simulink library "MAPH"  (R2016a)
settings: Solver=ode45  StartTime=0.0  StopTime=10.0  RelTol=1e-3
undefined symbols (not defined in the file): BUSY, CLEANED, EMPTY, FORWARD, ROB_EAST, ROB_NORTH, ROB_SOUTH, ROB_WEST, ROOM_SIDE_SIZE, UNCOVERED
settings Model: Creator=oelkawok  LastModifiedBy=omaro
settings DataIOCC: LimitDataPoints=on
settings DebuggingCC: AllowSymbolicDim=off

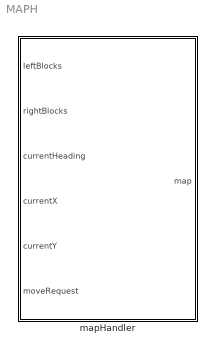
== system MAPH ==
  mapHandler : Subsystem

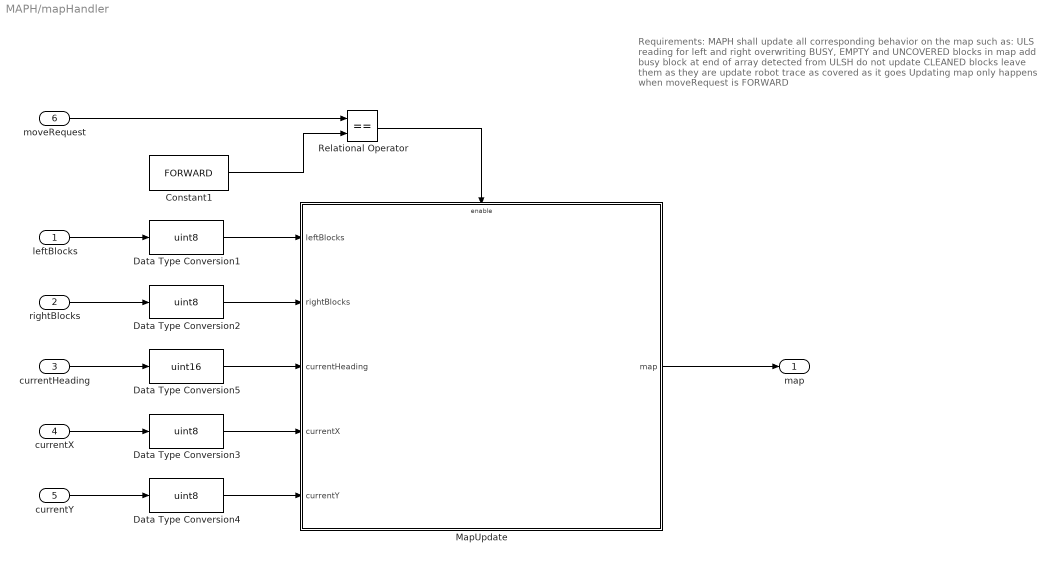
== system MAPH/mapHandler ==
  note: Requirements:
      | MAPH shall update all corresponding behavior on the map such as:
      | ULS reading for left and right
      | overwriting BUSY, EMPTY and UNCOVERED blocks in map
      | add busy block at end of array detected from ULSH
      | do not update CLEANED blocks leave them as they are
      | update robot trace as covered as it goes
      | Updating map only happens when moveRequest is FORWARD
  leftBlocks : Inport
  rightBlocks : Inport  Port=2
  currentHeading : Inport  Port=3
  currentX : Inport  Port=4
  currentY : Inport  Port=5
  moveRequest : Inport  Port=6
  Constant1 : Constant  Value=FORWARD
  Data Type Conversion{1..4} (4 alike) : DataTypeConversion  OutDataTypeStr=uint8
  Data Type Conversion5 : DataTypeConversion  OutDataTypeStr=uint16
  MapUpdate : Subsystem
  Relational Operator : RelationalOperator  Operator===  OutDataTypeStr=boolean
  map : Outport
  wires:
  Data Type Conversion1/1 -> MapUpdate/1(leftBlocks)
  Data Type Conversion2/1 -> MapUpdate/2(rightBlocks)
  Data Type Conversion3/1 -> MapUpdate/4(currentX)
  Data Type Conversion4/1 -> MapUpdate/5(currentY)
  Data Type Conversion5/1 -> MapUpdate/3(currentHeading)
  Relational Operator/1 -> MapUpdate/Enable
  moveRequest/1 -> Relational Operator/1
  Constant1/1 -> Relational Operator/2
  MapUpdate/1(map) -> map/1
  currentY/1 -> Data Type Conversion4/1
  currentX/1 -> Data Type Conversion3/1
  currentHeading/1 -> Data Type Conversion5/1
  rightBlocks/1 -> Data Type Conversion2/1
  leftBlocks/1 -> Data Type Conversion1/1

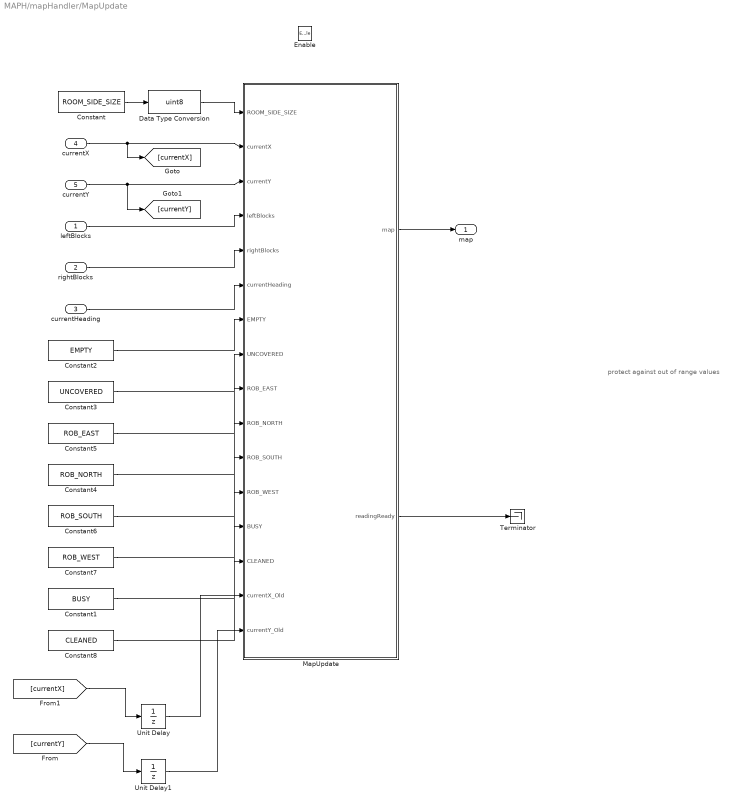
== system MAPH/mapHandler/MapUpdate ==
  note: protect against out of range values
  leftBlocks : Inport
  rightBlocks : Inport  Port=2
  currentHeading : Inport  Port=3
  currentX : Inport  Port=4
  currentY : Inport  Port=5
  Enable : EnablePort
  Constant : Constant  Value=ROOM_SIDE_SIZE
  Constant1 : Constant  Value=BUSY
  Constant2 : Constant  Value=EMPTY
  Constant3 : Constant  Value=UNCOVERED
  Constant4 : Constant  Value=ROB_NORTH
  Constant5 : Constant  Value=ROB_EAST
  Constant6 : Constant  Value=ROB_SOUTH
  Constant7 : Constant  Value=ROB_WEST
  Constant8 : Constant  Value=CLEANED
  Data Type Conversion : DataTypeConversion  OutDataTypeStr=uint8
  MapUpdate : Stateflow chart  TreatAsAtomicUnit=on
  Terminator : Terminator
  Unit Delay : UnitDelay  InitialCondition=10  SampleTime=-1
  Unit Delay1 : UnitDelay  InitialCondition=12  SampleTime=-1
  map : Outport
  wires:
  MapUpdate/1(map) -> map/1
  Unit Delay1/1 -> MapUpdate/16(currentY_Old)
  Unit Delay/1 -> MapUpdate/15(currentX_Old)
  [currentY] -> Unit Delay1/1
  [currentX] -> Unit Delay/1
  MapUpdate/2(readingReady) -> Terminator/1
  Constant2/1 -> MapUpdate/7(EMPTY)
  Constant8/1 -> MapUpdate/14(CLEANED)
  Constant3/1 -> MapUpdate/8(UNCOVERED)
  currentX/1 -> MapUpdate/2(currentX), [currentX]
  currentY/1 -> MapUpdate/3(currentY), [currentY]
  leftBlocks/1 -> MapUpdate/4(leftBlocks)
  rightBlocks/1 -> MapUpdate/5(rightBlocks)
  currentHeading/1 -> MapUpdate/6(currentHeading)
  Constant/1 -> Data Type Conversion/1
  Constant1/1 -> MapUpdate/13(BUSY)
  Data Type Conversion/1 -> MapUpdate/1(ROOM_SIDE_SIZE)
  Constant5/1 -> MapUpdate/9(ROB_EAST)
  Constant4/1 -> MapUpdate/10(ROB_NORTH)
  Constant6/1 -> MapUpdate/11(ROB_SOUTH)
  Constant7/1 -> MapUpdate/12(ROB_WEST)

== stateflow chart MAPH/mapHandler/MapUpdate/MapUpdate ==
  state MapUpdate
    state ULSHMapUpdate [parallel]
      settings: executionOrder=1
      state NorthCalc
        entry:
        leftCounter = 0;
        rightCounter = 0;
        startLeft = true;
        startRight = true;
        state ULSL [parallel]
          settings: executionOrder=2
          (history)
          state ULSL_Calc
          state Hit
          (junction 115) -> MapUpdate.ULSHMapUpdate.NorthCalc.ULSL.Hit [order 1] : [(leftCounter > leftBlocks)]
              | /map[currentX - leftCounter][currentY] = BUSY;
              | leftCounter = leftBlocks + 1;
              | startLeft = false;
          MapUpdate.ULSHMapUpdate.NorthCalc.ULSL.ULSL_Calc -> (junction 115) : [(leftCounter  <= leftBlocks)...
              | && ((currentX - leftCounter) > 0)]...
              | {leftCounter++;}
          (default) -> MapUpdate.ULSHMapUpdate.NorthCalc.ULSL.ULSL_Calc
          (junction 115) -> MapUpdate.ULSHMapUpdate.NorthCalc.ULSL.ULSL_Calc [order 2] : [map[currentX - leftCounter][currentY] != CLEANED]
              | /map[currentX - leftCounter][currentY] = EMPTY;
          MapUpdate.ULSHMapUpdate.NorthCalc.ULSL.Hit -> MapUpdate.ULSHMapUpdate.NorthCalc.ULSL.ULSL_Calc : [startLeft]/startLeft = false;
        state ULSR [parallel]
          settings: executionOrder=1
          (history)
          state ULSR_Calc
          state Hit
          MapUpdate.ULSHMapUpdate.NorthCalc.ULSR.ULSR_Calc -> (junction 56) : [(rightCounter  <= rightBlocks)...
              | && (rightCounter + currentX < ROOM_SIDE_SIZE)]...
              | {rightCounter++;}
          (default) -> MapUpdate.ULSHMapUpdate.NorthCalc.ULSR.ULSR_Calc
          (junction 56) -> MapUpdate.ULSHMapUpdate.NorthCalc.ULSR.Hit [order 1] : [(rightCounter > rightBlocks)]
              | /map[currentX + rightCounter][currentY] = BUSY;
              | rightCounter = rightBlocks + 1;
              | startRight = false;
          (junction 56) -> MapUpdate.ULSHMapUpdate.NorthCalc.ULSR.ULSR_Calc [order 2] : [map[currentX + rightCounter][currentY] != CLEANED]
              | /map[currentX + rightCounter][currentY] = EMPTY;
          MapUpdate.ULSHMapUpdate.NorthCalc.ULSR.Hit -> MapUpdate.ULSHMapUpdate.NorthCalc.ULSR.ULSR_Calc : [startRight]/startRight = false;
      state WestCalc
        entry:
        leftCounter = 0;
        rightCounter = 0;
        startLeft = true;
        startRight = true;
        state ULSL3 [parallel]
          settings: executionOrder=1
          (history)
          state ULSL_Calc
          state Hit
          MapUpdate.ULSHMapUpdate.WestCalc.ULSL3.ULSL_Calc -> (junction 236) : [(leftCounter  <= leftBlocks)...
              | && ((currentY + leftCounter) < ROOM_SIDE_SIZE)]...
              | {leftCounter++;}
          (default) -> MapUpdate.ULSHMapUpdate.WestCalc.ULSL3.ULSL_Calc
          (junction 236) -> MapUpdate.ULSHMapUpdate.WestCalc.ULSL3.Hit [order 1] : [(leftCounter > leftBlocks)]
              | /map[currentX][currentY + leftCounter] = BUSY;
              | leftCounter = leftBlocks + 1;
              | startLeft = false;
          (junction 236) -> MapUpdate.ULSHMapUpdate.WestCalc.ULSL3.ULSL_Calc [order 2] : [map[currentX][currentY + leftCounter] != CLEANED]
              | /map[currentX][currentY + leftCounter] = EMPTY;
          MapUpdate.ULSHMapUpdate.WestCalc.ULSL3.Hit -> MapUpdate.ULSHMapUpdate.WestCalc.ULSL3.ULSL_Calc : [startLeft]/startLeft = false;
        state ULSR3 [parallel]
          settings: executionOrder=2
          (history)
          state ULSR_Calc
          state Hit
            en:
          MapUpdate.ULSHMapUpdate.WestCalc.ULSR3.ULSR_Calc -> (junction 240) : [(rightCounter  <= rightBlocks)...
              | && (currentY - rightCounter > 0)]...
              | {rightCounter++;}
          (default) -> MapUpdate.ULSHMapUpdate.WestCalc.ULSR3.ULSR_Calc
          (junction 240) -> MapUpdate.ULSHMapUpdate.WestCalc.ULSR3.Hit [order 1] : [(rightCounter > rightBlocks)]
              | /map[currentX][currentY - rightCounter] = BUSY;
              | rightCounter = rightBlocks + 1;
              | startRight = false;
          (junction 240) -> MapUpdate.ULSHMapUpdate.WestCalc.ULSR3.ULSR_Calc [order 2] : [map[currentX][currentY - rightCounter] != CLEANED]
              | /map[currentX][currentY - rightCounter] = EMPTY;
          MapUpdate.ULSHMapUpdate.WestCalc.ULSR3.Hit -> MapUpdate.ULSHMapUpdate.WestCalc.ULSR3.ULSR_Calc : [startRight]/startRight = false;
      state Running
      state SouthCalc
        entry:
        leftCounter = 0;
        rightCounter = 0;
        startLeft = true;
        startRight = true;
        state ULSL1 [parallel]
          settings: executionOrder=1
          (history)
          state ULSL_Calc
          state Hit
          MapUpdate.ULSHMapUpdate.SouthCalc.ULSL1.ULSL_Calc -> (junction 196) : [(leftCounter  <= leftBlocks)...
              | && (rightCounter + currentX < ROOM_SIDE_SIZE)]...
              | {leftCounter++;}
          (default) -> MapUpdate.ULSHMapUpdate.SouthCalc.ULSL1.ULSL_Calc
          (junction 196) -> MapUpdate.ULSHMapUpdate.SouthCalc.ULSL1.Hit [order 1] : [(leftCounter > leftBlocks)]
              | /map[currentX + leftCounter][currentY] = BUSY;
              | leftCounter = leftBlocks + 1;
              | startLeft = false;
          (junction 196) -> MapUpdate.ULSHMapUpdate.SouthCalc.ULSL1.ULSL_Calc [order 2] : [map[currentX + leftCounter][currentY] != CLEANED]
              | /map[currentX + leftCounter][currentY] = EMPTY;
          MapUpdate.ULSHMapUpdate.SouthCalc.ULSL1.Hit -> MapUpdate.ULSHMapUpdate.SouthCalc.ULSL1.ULSL_Calc : [startLeft]/startLeft = false;
        state ULSR1 [parallel]
          settings: executionOrder=2
          (history)
          state ULSR_Calc
          state Hit
          MapUpdate.ULSHMapUpdate.SouthCalc.ULSR1.ULSR_Calc -> (junction 199) : [(rightCounter  <= rightBlocks)...
              | && (currentX - leftCounter) > 0]...
              | {rightCounter++;}
          (default) -> MapUpdate.ULSHMapUpdate.SouthCalc.ULSR1.ULSR_Calc
          (junction 199) -> MapUpdate.ULSHMapUpdate.SouthCalc.ULSR1.Hit [order 1] : [(rightCounter > rightBlocks)]
              | /map[currentX - rightCounter][currentY] = BUSY;
              | rightCounter = rightBlocks + 1;
              | startRight = false;
          (junction 199) -> MapUpdate.ULSHMapUpdate.SouthCalc.ULSR1.ULSR_Calc [order 2] : [map[currentX - rightCounter][currentY] != CLEANED]
              | /map[currentX - rightCounter][currentY] = EMPTY;
          MapUpdate.ULSHMapUpdate.SouthCalc.ULSR1.Hit -> MapUpdate.ULSHMapUpdate.SouthCalc.ULSR1.ULSR_Calc : [startRight]/startRight = false;
      state EastCalc
        entry:
        leftCounter = 0;
        rightCounter = 0;
        startLeft = true;
        startRight = true;
        state ULSL2 [parallel]
          settings: executionOrder=1
          (history)
          state ULSL_Calc
          state Hit
          MapUpdate.ULSHMapUpdate.EastCalc.ULSL2.ULSL_Calc -> (junction 212) : [(leftCounter  <= leftBlocks)...
              | && ((currentY - leftCounter) > 0)]...
              | {leftCounter++;}
          (junction 212) -> MapUpdate.ULSHMapUpdate.EastCalc.ULSL2.Hit [order 1] : [(leftCounter > leftBlocks)]
              | /map[currentX][currentY - leftCounter] = BUSY;
              | leftCounter = leftBlocks + 1;
              | startLeft = false;
          (default) -> MapUpdate.ULSHMapUpdate.EastCalc.ULSL2.ULSL_Calc
          (junction 212) -> MapUpdate.ULSHMapUpdate.EastCalc.ULSL2.ULSL_Calc [order 2] : [(map[currentX][currentY - leftCounter] != CLEANED)]
              | /map[currentX][currentY - leftCounter] = EMPTY;
          MapUpdate.ULSHMapUpdate.EastCalc.ULSL2.Hit -> MapUpdate.ULSHMapUpdate.EastCalc.ULSL2.ULSL_Calc : [startLeft]/startLeft = false;
        state ULSR2 [parallel]
          settings: executionOrder=2
          (history)
          state ULSR_Calc
          state Hit
          MapUpdate.ULSHMapUpdate.EastCalc.ULSR2.ULSR_Calc -> (junction 208) : [(rightCounter  <= rightBlocks)...
              | && (rightCounter + currentY < ROOM_SIDE_SIZE)]...
              | {rightCounter++;}
          (default) -> MapUpdate.ULSHMapUpdate.EastCalc.ULSR2.ULSR_Calc
          (junction 208) -> MapUpdate.ULSHMapUpdate.EastCalc.ULSR2.Hit [order 1] : [(rightCounter > rightBlocks)]
              | /map[currentX][currentY + rightCounter] = BUSY;
              | rightCounter = rightBlocks + 1;
              | startRight = false;
          (junction 208) -> MapUpdate.ULSHMapUpdate.EastCalc.ULSR2.ULSR_Calc [order 2] : [(map[currentX][currentY + rightCounter] != CLEANED)]
              | /map[currentX][currentY + rightCounter] = EMPTY;
          MapUpdate.ULSHMapUpdate.EastCalc.ULSR2.Hit -> MapUpdate.ULSHMapUpdate.EastCalc.ULSR2.ULSR_Calc : [startRight]/startRight = false;
      (default) -> Running
      Running -> WestCalc [order 1] : [(currentHeading == ROB_WEST) ...
          | && (hasChanged(currentHeading)...
          | || hasChanged(currentX))]
          | /readingReady = false;
      Running -> NorthCalc [order 4] : [(currentHeading == ROB_NORTH) ...
          | && (hasChanged(currentHeading)...
          | || hasChanged(currentY))]
      (junction 165) -> Running : [(leftCounter > leftBlocks)...
          |  &&(rightCounter > rightBlocks)]
          | /readingReady = true;
      WestCalc -> (junction 165)
      EastCalc -> (junction 165)
      NorthCalc -> (junction 118)
      (junction 118) -> Running : [((leftCounter > leftBlocks)...
          |  &&(rightCounter > rightBlocks))...
          | || hasChanged(currentHeading)]
          | /readingReady = true;
      SouthCalc -> (junction 118)
      Running -> EastCalc [order 2] : [(currentHeading == ROB_EAST) ...
          | && (hasChanged(currentHeading)...
          | || hasChanged(currentX))]
          | /readingReady = false;
      Running -> SouthCalc [order 3] : [(currentHeading == ROB_SOUTH) ...
          | && (hasChanged(currentHeading)...
          | || hasChanged(currentY))]
          | /readingReady = false;
    state updateRobotTrace [parallel]
      settings: executionOrder=2
      state Idle
      state updateX
        en:
        map[currentX_Old][currentY] = CLEANED;
      state updateY
        en:
        map[currentX][currentY_Old] = CLEANED;
      (default) -> Idle
      updateX -> Idle
      updateY -> Idle
      Idle -> (junction 288)
      (junction 288) -> updateX [order 1] : [hasChanged(currentX)]
      (junction 288) -> updateY [order 2] : [hasChanged(currentY)]
  (default) -> MapUpdate
  data: map output uint8 size=[ROOM_SIDE_SIZE ROOM_SIDE_SIZE] =map; ROOM_SIDE_SIZE input uint8; currentX input uint8; currentY input uint8; leftBlocks input; rightBlocks input; currentHeading input; readingReady output double; leftCounter local uint8; rightCounter local uint8; startLeft local boolean; startRight local boolean; EMPTY input; UNCOVERED input; ROB_EAST input; ROB_NORTH input; ROB_SOUTH input; ROB_WEST input; BUSY input; CLEANED input; currentX_Old input; currentY_Old input
